simulink model "T50_VD"  (R2016b)
settings: configuration reference "CodeGenConfigSet" (kept outside this file)
values from neighbouring files (symbols this model uses):
  DDRC_DurDebT50_tiErrDebDef_C = Calibration.Parameter    [init_T50_VD.m]    (also in init_T50_VD_SIL.m = Simulink.Parameter)
  DDRC_DurDebT50_tiErrDebOk_C = Calibration.Parameter    [init_T50_VD.m]    (also in init_T50_VD_SIL.m = Simulink.Parameter)
  T50_tiEmgcyReq_C = Calibration.Parameter    [init_T50_VD.m]    (also in init_T50_VD_SIL.m = Simulink.Parameter)
undefined symbols (not defined in the file or in its folder): T50_VD_DT
libraries: CXLib x4
settings Model: Creator=xuxingpei  LastModifiedBy=xuxingpei
settings ConfigSetRef: SourceLocation=Base Workspace

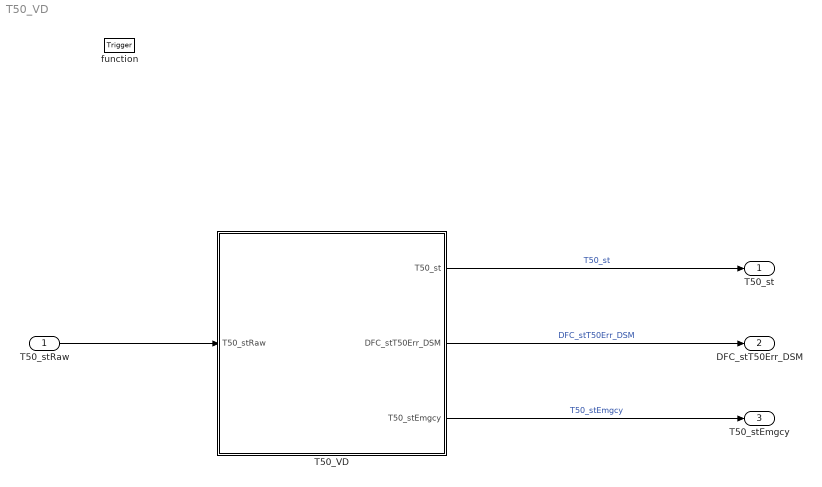
== system T50_VD ==
  T50_stRaw : Inport  Description=Terminal 50 status after debouncing  OutDataTypeStr=Enum: Switch_conv
  function : TriggerPort  TriggerType=function-call  VariantControl=Variant
  T50_VD : Subsystem
  T50_st : Outport  Description=Terminal 50 status after Check  OutDataTypeStr=Enum: Switch_conv
  DFC_stT50Err_DSM : Outport  Description=Terminal 50 status after DSM  Port=2  OutMin=0  OutMax=1  OutDataTypeStr=boolean
  T50_stEmgcy : Outport  Description=Terminal 50 status after debouncing  Port=3  OutMin=0  OutMax=1  OutDataTypeStr=boolean
  wires:
  T50_VD/1(T50_st) -> T50_st/1  "T50_st"
  T50_VD/2(DFC_stT50Err_DSM) -> DFC_stT50Err_DSM/1  "DFC_stT50Err_DSM"
  T50_stRaw/1 -> T50_VD/1(T50_stRaw)
  T50_VD/3(T50_stEmgcy) -> T50_stEmgcy/1  "T50_stEmgcy"

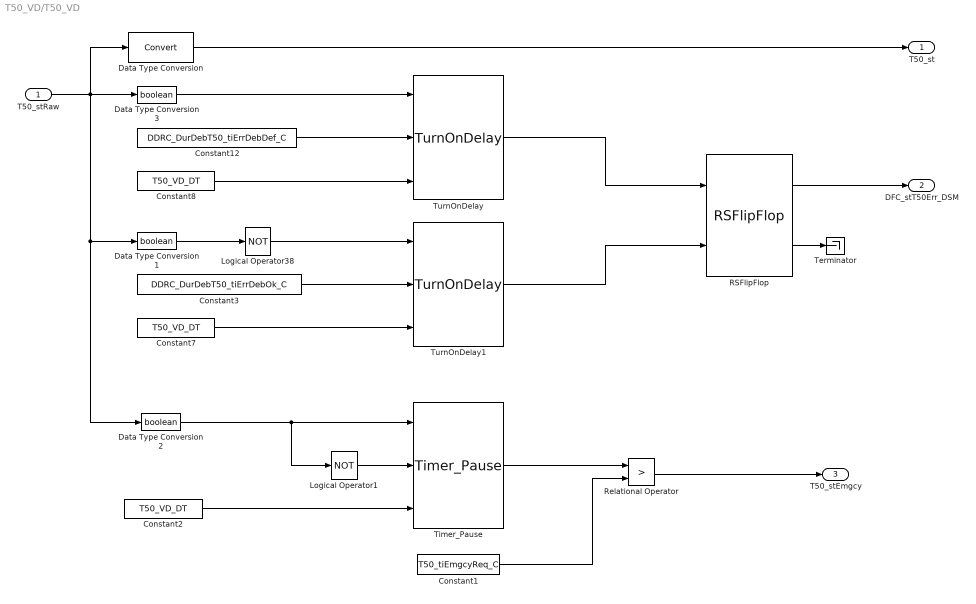
== system T50_VD/T50_VD ==
  T50_stRaw : Inport
  Constant1 : Constant  Value=T50_tiEmgcyReq_C
  Constant12 : Constant  Value=DDRC_DurDebT50_tiErrDebDef_C
  Constant2 : Constant  Value=T50_VD_DT
  Constant3 : Constant  Value=DDRC_DurDebT50_tiErrDebOk_C
  Constant7 : Constant  Value=T50_VD_DT
  Constant8 : Constant  Value=T50_VD_DT
  Data Type Conversion : DataTypeConversion
  Data Type Conversion1 : DataTypeConversion  OutDataTypeStr=boolean
  Data Type Conversion2 : DataTypeConversion  OutDataTypeStr=boolean
  Data Type Conversion3 : DataTypeConversion  OutDataTypeStr=boolean
  Logical Operator1 : Logic  Operator=NOT  AllPortsSameDT=off  OutDataTypeStr=boolean
  Logical Operator38 : Logic  Operator=NOT  AllPortsSameDT=off  OutDataTypeStr=boolean
  RSFlipFlop : CXLib/RSFlipFlop
  Relational Operator : RelationalOperator  Operator=>  OutDataTypeStr=boolean  RndMeth=Simplest
  Terminator : Terminator
  Timer_Pause : CXLib/Timer_Pause
  TurnOnDelay : CXLib/TurnOnDelay
  TurnOnDelay1 : CXLib/TurnOnDelay
  T50_st : Outport
  DFC_stT50Err_DSM : Outport  Description=Terminal 50 status after DSM  Port=2  OutMin=0  OutMax=1  OutDataTypeStr=boolean
  T50_stEmgcy : Outport  Port=3
  wires:
  Constant7/1 -> TurnOnDelay1/3
  RSFlipFlop/1 -> DFC_stT50Err_DSM/1
  Constant8/1 -> TurnOnDelay/3
  TurnOnDelay1/1 -> RSFlipFlop/2
  Constant12/1 -> TurnOnDelay/2
  Constant3/1 -> TurnOnDelay1/2
  TurnOnDelay/1 -> RSFlipFlop/1
  Logical Operator38/1 -> TurnOnDelay1/1
  RSFlipFlop/2 -> Terminator/1
  Data Type Conversion3/1 -> TurnOnDelay/1
  Data Type Conversion1/1 -> Logical Operator38/1
  T50_stRaw/1 -> Data Type Conversion/1, Data Type Conversion3/1, Data Type Conversion1/1, Data Type Conversion2/1
  Timer_Pause/1 -> Relational Operator/1
  Constant1/1 -> Relational Operator/2
  Relational Operator/1 -> T50_stEmgcy/1
  Data Type Conversion2/1 -> Logical Operator1/1, Timer_Pause/1
  Data Type Conversion/1 -> T50_st/1
  Constant2/1 -> Timer_Pause/3
  Logical Operator1/1 -> Timer_Pause/2
